simulink model "RL_GHV_open_smc"  (R2023b)
settings: Solver=VariableStepAuto  StartTime=0  StopTime=840  FixedStep=0.0000001  MaxStep=0.001  RelTol=1e-3
InitFcn:
  | run('init.m')
values from neighbouring files (symbols this model uses):
  GHV_cfg = struct()    [GHV_Configuration.m]
libraries: simulink_extras x4, aerolibasang x3, aerolibtransform2 x2, aerolib6dof2 x1, aerolibatmos2 x1, matrix_library x1, aerolibgravity2 x1, rllib x1
settings Model: Creator=Admin  LastModifiedBy=Admin
settings SolverCC: AllowMultiTaskInputOutput=on  ZeroCrossControl=EnableAll  ZeroCrossAlgorithm=Adaptive  AutoInsertRateTranBlk=on
settings DebuggingCC: IgnoredZcDiagnostic=none

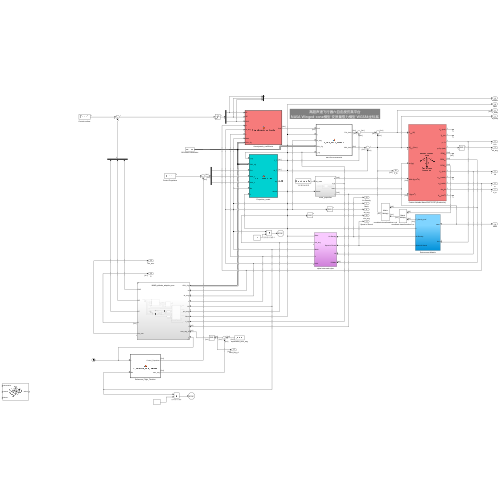
[thumbnail: Simulink's stored preview of the top-level diagram]
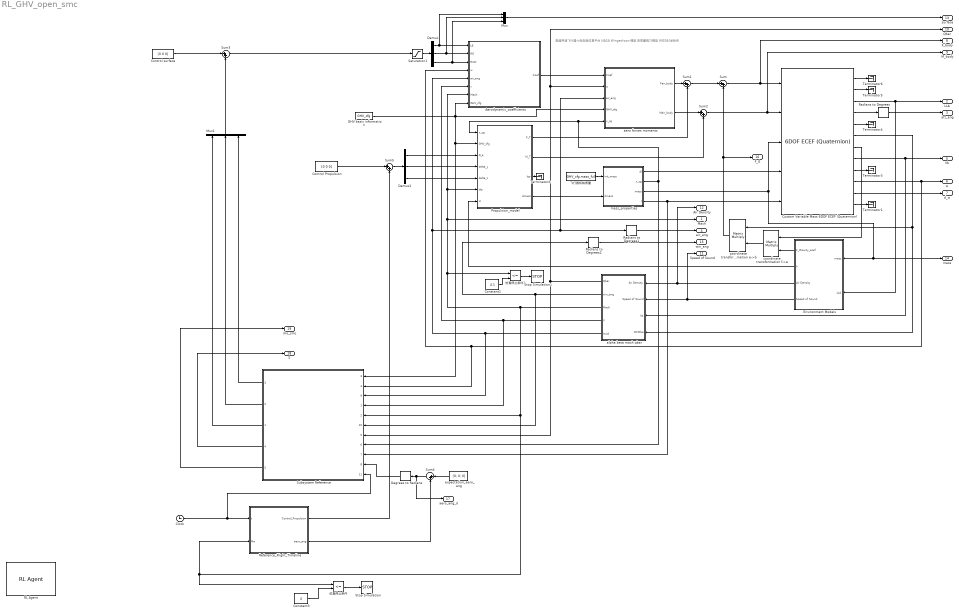
== system RL_GHV_open_smc ==
  note: 高超声速飞行器六自由度仿真平台
      | NASA Winged-cone模型 变质量推力模型 WGS84坐标系
  Aerodynamic_coefficients : MATLAB Function  TreatAsAtomicUnit=on
  Clock : Clock
  Constant1 : Constant  Value=4.1
  Constant3 : Constant  Value=4
  Control Propulsion : Constant  Value=[0 0 0]
  Control surface : Constant  Value=[0 0 0]
  Custom Variable Mass 6DOF ECEF (Quaternion) : aerolib6dof2/6DOF ECEF (Quaternion)  units=Metric (MKS)  mtype=Custom Variable  xg_0=LLA_init  Vm_0=Speed_init  eul_0=Euler_init  pm_0=Omega_init  mass_0=1.0  mass_e=0.5  mass_f=2.0  inertia=eye(3)  inertia_e=eye(3)  inertia_f=2*eye(3)  vre_flag=off  abi_flag=off  ptype=Custom  R=6378137  F=1/298.257223563  w_E=0  angle_in=Internal  LPM0=0  quat_statename=''  pm_statename=''  Vm_statename=''  posfixedframe_statename=''  posinertial_statename=''  LPM_statename=''  mass_statename=''
      settings: LibrarySourceBlock=|
      | aerolib6dof2/Custom Variable Mass 6DOF
      | ECEF (Quaternion)
  Degrees to Radians : simulink_extras/Transformations/Degrees to Radians
  Demux : Demux  Outputs=3
  Demux1 : Demux  Outputs=3
  Environment Models : Subsystem
  GHV basic information : Constant  Value=GHV_cfg  VectorParams1D=off  OutDataTypeStr=Bus: slBus1
  Mux : Mux  Inputs=3
  Mux1 : Mux  Inputs=3
  Propulsion_model : MATLAB Function  TreatAsAtomicUnit=on
  RL Agent : rllib/RL Agent  Agent=agentObj  ExternalActionAsInput=off  ProvideLastAction=off  ProvideCumRwd=off  TreatAsDirectFeedthrough=on  UseStrictObservationDataTypes=on
  Radians to Degrees : simulink_extras/Transformations/Radians to Degrees
  Radians to Degrees1 : simulink_extras/Transformations/Radians to Degrees
  Radians to Degrees2 : simulink_extras/Transformations/Radians to Degrees
  Reference_Flight_Timeline : MATLAB Function  TreatAsAtomicUnit=on
  Saturation1 : Saturate  UpperLimit=30  LowerLimit=-30
  Stop Simulation : Stop
  Stop Simulation1 : Stop
  Subsystem Reference : Subsystem  ReferencedSubsystem=MIMO_attitude_adaptive_smc
      settings: PortSchema="{\"entries\":[{\"content\":{\"sides\":[{\"content\":{\"connectorIds\":[\"In3\",\"In4\",\"In9\",\"In1\",\"In2\",\"In10\",\"In5\",\"In6\",\"In7\",\"In8\",\"In11\"]},\"type\":\"ConnectorPlacement.EquallySpacedRectSide\",\"uuid\":\"d16573b0-003d-4406-8236-24f2e66cdcc6\"},{\"content\":{\"connectorIds\":[\"Out3\",\"Out2\",\"Out1\",\"Out4\",\"Out5\"],\"side\":\"RIGHT\"},\"type\":\"ConnectorPlacement.EquallySpacedRectSide\",\"uuid\":\"8f215ada-bc58-4b5c-bd2e-12efaced2d85\"},{\"content\":{\"side\":\"TOP\"},\"type\":\"ConnectorPlacement.EquallySpacedRectSide\",\"uuid\":\"754feef1-e2fd-4717-9f83-2c281c09523f\"}]},\"type\":\"ConnectorPlacement.EquallySpacedConnector\",\"uuid\":\"c4c9c765-2f71-4497-9966-89bfbf2bbd3f\"}],\"packageUris\":[\"http://schema.mathworks.com/mf0/Connector/R2020b\"],\"version\":\"1.0\"}"
  Sum{,1..5} (6 alike) : Sum  Inputs=|++
  Terminator{1..6} (6 alike) : Terminator
  aero forces moments : MATLAB Function  TreatAsAtomicUnit=on
  alpha beta mach qbar : Subsystem
  coordinate transformation e->b : Product  Multiplication=Matrix(*)
  coordinate transformation f->e : Product  Multiplication=Matrix(*)
  expectation_aero_ang : Constant  Value=[0; 0; 0]  VectorParams1D=off
  mass_properties : Subsystem
  仿真停止条件 : RelationalOperator  Operator=<=  OutDataTypeStr=boolean  RndMeth=Simplest  InputSameDT=off
  仿真停止条件1 : RelationalOperator  Operator=<=  OutDataTypeStr=boolean  RndMeth=Simplest  InputSameDT=off
  飞行器初始质量 : Constant  Value=GHV_cfg.mass_full
  Mach : Outport
  LLA : Outport  Port=2
  att_ang : Outport  Port=3
  air_ang : Outport  Port=4
  Vb : Outport  Port=5
  w : Outport  Port=6
  d_w : Outport  Port=7
  F_body : Outport  Port=8
  M_body : Outport  Port=9
  Qbar : Outport  Port=10
  Speed of Sound : Outport  Port=11
  Air Density : Outport  Port=12
  surface : Outport  Port=13
  mass : Outport  Port=14
  win_ang : Outport  Port=15
  F_G : Outport  Port=16
  aero_ang_d : Outport  Port=17
  S : Outport  Port=18
  rho_smc : Outport  Port=19
  wires:
  Control surface/1 -> Sum3/1
  Degrees to Radians/1 -> Subsystem Reference/8
  Subsystem Reference/1 -> Mux1/1
  Subsystem Reference/2 -> Mux1/2
  Subsystem Reference/3 -> Mux1/3
  coordinate transformation e->b/1 -> F_G/1, Sum/2
  Aerodynamic_coefficients/1(Coef) -> aero forces moments/1(Coef)
  mass_properties/2(x_cg) -> Propulsion_model/1(x_cg), aero forces moments/5(x_cg), Subsystem Reference/6
  coordinate transformation f->e/1 -> coordinate transformation e->b/2
  飞行器初始质量/1 -> mass_properties/1(init_mass)
  Radians to Degrees1/1 -> air_ang/1
  Propulsion_model/2(M_T) -> Sum2/2
  Custom Variable Mass 6DOF ECEF (Quaternion)/1 -> Terminator6/1
  Custom Variable Mass 6DOF ECEF (Quaternion)/9 -> Terminator3/1
  mass_properties/3(mass) -> Environment Models/1(mass), mass/1, Custom Variable Mass 6DOF ECEF (Quaternion)/3
  Radians to Degrees2/1 -> win_ang/1
  Demux/1 -> Aerodynamic_coefficients/1(LE), Mux/1
  Custom Variable Mass 6DOF ECEF (Quaternion)/5 -> Terminator4/1
  Saturation1/1 -> Demux/1
  Demux1/2 -> Propulsion_model/4(delta_y)
  Control Propulsion/1 -> Sum5/1
  Propulsion_model/1(F_T) -> Sum1/2
  Custom Variable Mass 6DOF ECEF (Quaternion)/3 -> LLA/1, Environment Models/2(LLA)
  Demux/2 -> Aerodynamic_coefficients/2(RE), Mux/2
  alpha beta mach qbar/5(Incid) -> aero forces moments/3(air_ang), Radians to Degrees1/1, Aerodynamic_coefficients/5(air_ang), Subsystem Reference/9
  Sum2/1 -> M_body/1, Custom Variable Mass 6DOF ECEF (Quaternion)/2
  Propulsion_model/4(dmass) -> mass_properties/2(dmass)
  Sum1/1 -> Sum/1
  Environment Models/3(Air Density) -> alpha beta mach qbar/1(Air Density), Air Density/1
  Environment Models/2(h) -> Propulsion_model/7(H)
  alpha beta mach qbar/1(Qbar) -> Subsystem Reference/5, aero forces moments/2(q), Qbar/1
  aero forces moments/1(Fair_body) -> Sum1/1
  Radians to Degrees/1 -> att_ang/1
  Custom Variable Mass 6DOF ECEF (Quaternion)/6 -> alpha beta mach qbar/4(DCMbe), coordinate transformation e->b/1
  aero forces moments/2(Mair_body) -> Sum2/1
  Demux1/3 -> Propulsion_model/5(delta_z)
  Custom Variable Mass 6DOF ECEF (Quaternion)/10 -> w/1, Aerodynamic_coefficients/4(w), Subsystem Reference/4
  Mux/1 -> surface/1
  GHV basic information/1 -> Subsystem Reference/3, Propulsion_model/2(GHV_cfg), aero forces moments/4(GHV_cfg), Aerodynamic_coefficients/8(GHV_cfg)
  Demux/3 -> Aerodynamic_coefficients/3(RUD), Mux/3
  alpha beta mach qbar/2(win_ang) -> Radians to Degrees2/1, Subsystem Reference/10
  Sum3/1 -> Saturation1/1
  Propulsion_model/3(Isp) -> Terminator2/1
  Environment Models/1(F_Gravity_ecef) -> coordinate transformation f->e/2
  Custom Variable Mass 6DOF ECEF (Quaternion)/11 -> d_w/1
  Demux1/1 -> Propulsion_model/3(PLA)
  mass_properties/1(dI) -> Custom Variable Mass 6DOF ECEF (Quaternion)/4
  Custom Variable Mass 6DOF ECEF (Quaternion)/7 -> coordinate transformation f->e/1
  Custom Variable Mass 6DOF ECEF (Quaternion)/2 -> Terminator5/1
  Custom Variable Mass 6DOF ECEF (Quaternion)/8 -> Vb/1, alpha beta mach qbar/3(Vb)
  alpha beta mach qbar/4(V) -> Aerodynamic_coefficients/6(v), Subsystem Reference/1
  Environment Models/4(Speed of Sound) -> alpha beta mach qbar/2(Speed of Sound), Speed of Sound/1
  Custom Variable Mass 6DOF ECEF (Quaternion)/12 -> Terminator1/1
  Custom Variable Mass 6DOF ECEF (Quaternion)/4 -> Radians to Degrees/1
  Sum/1 -> F_body/1, Custom Variable Mass 6DOF ECEF (Quaternion)/1
  mass_properties/4(I) -> Custom Variable Mass 6DOF ECEF (Quaternion)/5, Subsystem Reference/7
  expectation_aero_ang/1 -> Sum4/1
  Reference_Flight_Timeline/2(aero_ang) -> Sum4/2
  Sum5/1 -> Demux1/1
  Reference_Flight_Timeline/1(Control_Propulsion) -> Sum5/2
  Clock/1 -> Reference_Flight_Timeline/1(t), Subsystem Reference/11
  仿真停止条件/1 -> Stop Simulation/1
  Constant3/1 -> 仿真停止条件/2
  alpha beta mach qbar/3(Mach) -> 仿真停止条件1/1, Mach/1, Propulsion_model/6(Ma), Aerodynamic_coefficients/7(Mach), Reference_Flight_Timeline/2(Ma), 仿真停止条件/1, Subsystem Reference/2
  Sum4/1 -> aero_ang_d/1, Degrees to Radians/1
  Subsystem Reference/4 -> S/1
  Mux1/1 -> Sum3/2
  Subsystem Reference/5 -> rho_smc/1
  Constant1/1 -> 仿真停止条件1/2
  仿真停止条件1/1 -> Stop Simulation1/1

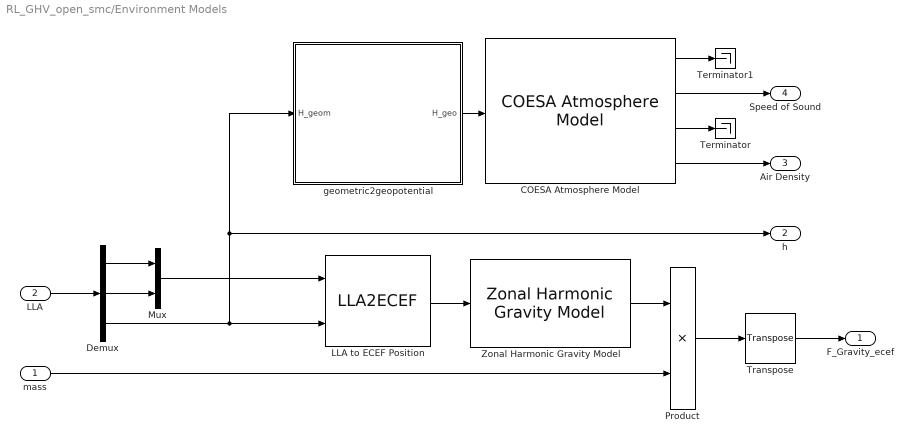
== system RL_GHV_open_smc/Environment Models ==
  mass : Inport
  LLA : Inport  Port=2
  COESA Atmosphere Model : aerolibatmos2/COESA Atmosphere Model  units=Metric (MKS)  spec=1976 COESA-extended U.S. Standard Atmosphere  model=Profile  profile_var=High temperature  profile_percent=1%  profile_alt=5 km (16404 ft)  envelope_var=High temperature  envelope_percent=1%  action=Warning
  Demux : Demux  Outputs=3
  LLA to ECEF Position : LLA2ECEF
  Mux : Mux  Inputs=2
  Product : Product
  Terminator : Terminator
  Terminator1 : Terminator
  Transpose : matrix_library/Transpose
  Zonal Harmonic Gravity Model : aerolibgravity2/Zonal Harmonic Gravity Model  units=Metric (MKS)  degree=2  action=Warning  ptype=Earth  R=6378136.3  GM=398600441500000  jvalue=[1.0826269e-03 -2.5323000e-06 -1.6204000e-06]
  geometric2geopotential : MATLAB Function  TreatAsAtomicUnit=on
  F_Gravity_ecef : Outport
  h : Outport  Port=2
  Air Density : Outport  Port=3
  Speed of Sound : Outport  Port=4
  wires:
  COESA Atmosphere Model/1 -> Terminator1/1
  COESA Atmosphere Model/2 -> Speed of Sound/1
  COESA Atmosphere Model/3 -> Terminator/1
  COESA Atmosphere Model/4 -> Air Density/1
  LLA to ECEF Position/1 -> Zonal Harmonic Gravity Model/1
  Mux/1 -> LLA to ECEF Position/1
  Demux/3 -> h/1, geometric2geopotential/1(H_geom), LLA to ECEF Position/2
  Demux/1 -> Mux/1
  Demux/2 -> Mux/2
  LLA/1 -> Demux/1
  mass/1 -> Product/2
  Zonal Harmonic Gravity Model/1 -> Product/1
  Product/1 -> Transpose/1
  Transpose/1 -> F_Gravity_ecef/1
  geometric2geopotential/1(H_geo) -> COESA Atmosphere Model/1

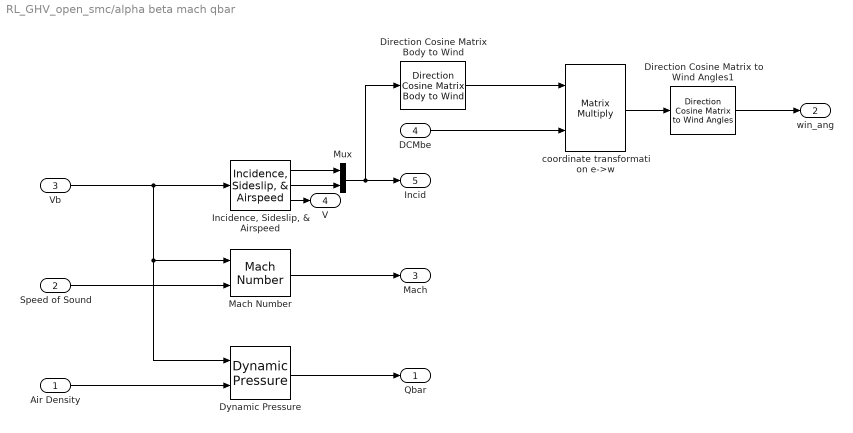
== system RL_GHV_open_smc/alpha beta mach qbar ==
  Air Density : Inport
  Speed of Sound : Inport  Port=2
  Vb : Inport  Port=3
  DCMbe : Inport  Port=4
  Direction Cosine Matrix Body to Wind : aerolibtransform2/Direction Cosine Matrix Body to Wind
  Direction Cosine Matrix to Wind Angles1 : aerolibtransform2/Direction Cosine Matrix to Wind Angles  action=None  tolerance=eps(2)
  Dynamic Pressure : aerolibasang/Dynamic Pressure
  "Incidence, Sideslip, & Airspeed" : aerolibasang/Incidence, Sideslip, & Airspeed
  Mach Number : aerolibasang/Mach Number
  Mux : Mux  Inputs=2
  coordinate transformation e->w : Product  Multiplication=Matrix(*)
  Qbar : Outport
  win_ang : Outport  Port=2
  Mach : Outport  Port=3
  V : Outport  Port=4
  Incid : Outport  Port=5
  wires:
  Speed of Sound/1 -> Mach Number/2
  Mach Number/1 -> Mach/1
  "Incidence, Sideslip, & Airspeed"/2 -> Mux/2
  Vb/1 -> Dynamic Pressure/1, Mach Number/1, "Incidence, Sideslip, & Airspeed"/1
  Dynamic Pressure/1 -> Qbar/1
  Mux/1 -> Direction Cosine Matrix Body to Wind/1, Incid/1
  "Incidence, Sideslip, & Airspeed"/1 -> Mux/1
  Air Density/1 -> Dynamic Pressure/2
  "Incidence, Sideslip, & Airspeed"/3 -> V/1
  DCMbe/1 -> coordinate transformation e->w/2
  Direction Cosine Matrix Body to Wind/1 -> coordinate transformation e->w/1
  coordinate transformation e->w/1 -> Direction Cosine Matrix to Wind Angles1/1
  Direction Cosine Matrix to Wind Angles1/1 -> win_ang/1

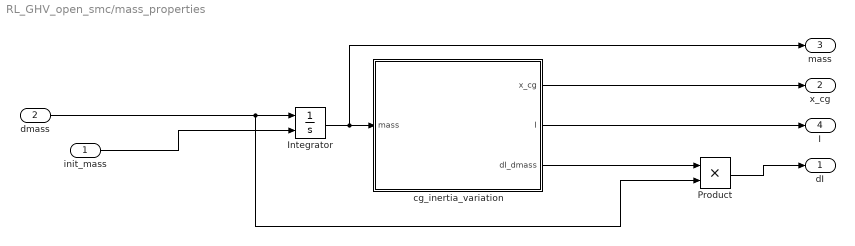
== system RL_GHV_open_smc/mass_properties ==
  init_mass : Inport
  dmass : Inport  Port=2
  Integrator : Integrator  InitialConditionSource=external
  Product : Product
  cg_inertia_variation : MATLAB Function  TreatAsAtomicUnit=on
  dI : Outport
  x_cg : Outport  Port=2
  mass : Outport  Port=3
  I : Outport  Port=4
  wires:
  Integrator/1 -> mass/1, cg_inertia_variation/1(mass)
  init_mass/1 -> Integrator/2
  cg_inertia_variation/3(dI_dmass) -> Product/1
  dmass/1 -> Product/2, Integrator/1
  cg_inertia_variation/2(I) -> I/1
  cg_inertia_variation/1(x_cg) -> x_cg/1
  Product/1 -> dI/1

== matlab function RL_GHV_open_smc/Propulsion_model ==
  data: F_T output; M_T output; x_cg input; GHV_cfg input; PLA input; delta_y input; delta_z input; Ma input; H input; Isp output; dmass output
function [F_T,M_T, Isp,  dmass] = S_Propulsion_model(x_cg, GHV_cfg, PLA, delta_y, delta_z, Ma, H)
    F_T = zeros(3, 1); %#ok<PREALL>
    M_T = zeros(3, 1); %#ok<PREALL>
   [F_T, M_T, Isp, dmass] = Propulsion_model(PLA, H, Ma, delta_y, delta_z, GHV_cfg, x_cg);

end

== matlab function RL_GHV_open_smc/Aerodynamic_coefficients ==
  data: LE input; Coef output; RE input; RUD input; w input; air_ang input; v input; Mach input; GHV_cfg input
function Coef = S_Aerodynamic_coefficients(LE, RE, RUD, w, air_ang,v, Mach, GHV_cfg)
    Coef = zeros(6, 1);
    Coef = Aerodynamic_coefficients(LE, RE, RUD, air_ang, v, w, Mach, GHV_cfg);

end

== matlab function RL_GHV_open_smc/aero forces moments ==
  data: Coef input; q input; air_ang input; GHV_cfg input; x_cg input; Fair_body output; Mair_body output
function [Fair_body, Mair_body] = S_aero_forces_moments(Coef, q, air_ang, GHV_cfg, x_cg)

    Fair_body = zeros(3, 1); %#ok<PREALL>
    Mair_body = zeros(3, 1); %#ok<PREALL>
    [Fair_body, Mair_body] = aero_forces_moments(Coef, q, GHV_cfg, x_cg, air_ang);

end

== matlab function RL_GHV_open_smc/Environment Models/geometric2geopotential ==
  data: H_geom input; H_geo output
function H_geo = S_geometric2geopotential(H_geom)

    H_geo = geometric2geopotential(H_geom);

end

== matlab function RL_GHV_open_smc/mass_properties/cg_inertia_variation ==
  data: mass input; x_cg output; I output; dI_dmass output
function [x_cg, I, dI_dmass] = S_cg_inertia_variation(mass)

     [x_cg, I, dI_dmass] = cg_inertia_variation(mass);
     
end

== matlab function RL_GHV_open_smc/Reference_Flight_Timeline ==
  data: Control_Propulsion output; t input; aero_ang output; Ma input
function [Control_Propulsion,aero_ang] = S_Reference_Flight_Timeline(t, Ma)

   [aero_ang, Control_Propulsion] = Reference_Flight_Timeline(t, Ma);

end
